simulink model "task4_rfj"  (R2022b)
settings: Solver=VariableStepAuto  StartTime=0.0  StopTime=param.T  FixedStep=0.01  MaxStep=0.01  RelTol=1e-3
undefined symbols (not defined in the file or in its folder): param
settings Model: Creator=15043  LastModifiedBy=15043
settings SolverCC: AlgebraicLoopSolver=TrustRegion
settings DebuggingCC: ArithmeticOperatorsInVariantConditions=warning
settings SFSimCC: CustomCodeUndefinedFunction=UseInterfaceOnly

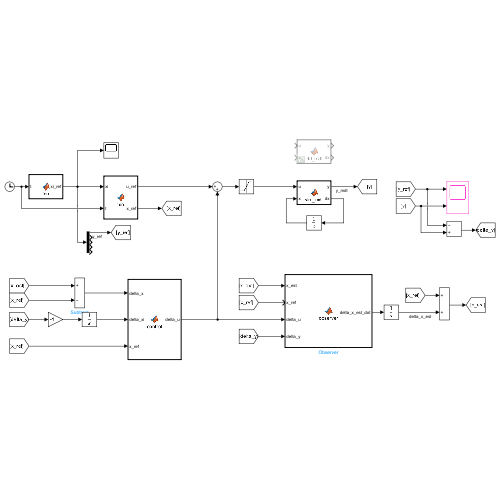
[thumbnail: Simulink's stored preview of the top-level diagram]
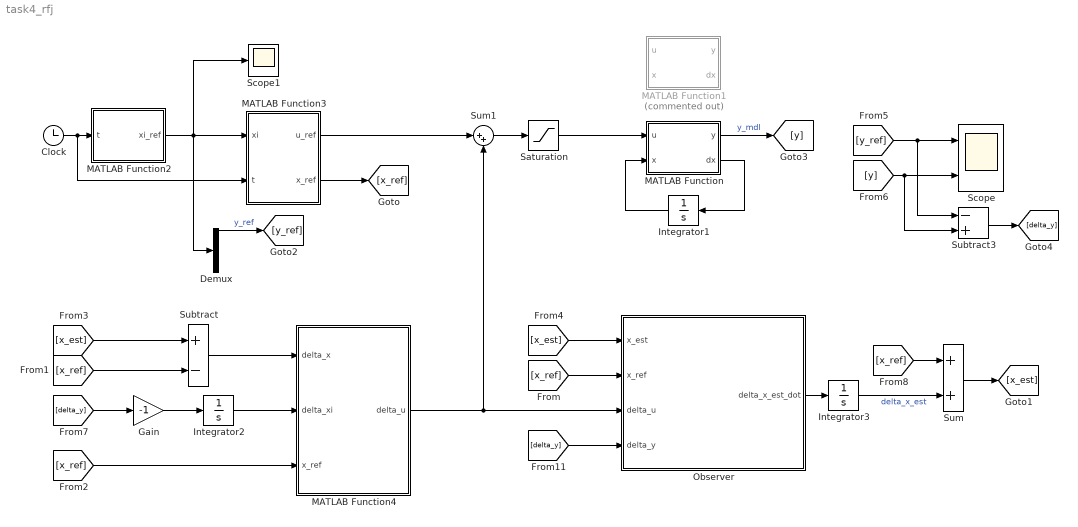
== system task4_rfj ==
  Clock : Clock
  Demux : Demux  Outputs=5
  Gain : Gain  Gain=-1
  Integrator1 : Integrator  InitialCondition=param.x0
  Integrator2 : Integrator
  Integrator3 : Integrator  InitialCondition=param.delta_x_est0
  MATLAB Function : MATLAB Function  TreatAsAtomicUnit=on
  MATLAB Function1 : MATLAB Function  Commented=on  TreatAsAtomicUnit=on
  MATLAB Function2 : MATLAB Function  TreatAsAtomicUnit=on
  MATLAB Function3 : MATLAB Function  TreatAsAtomicUnit=on
  MATLAB Function4 : MATLAB Function  TreatAsAtomicUnit=on
  Observer : MATLAB Function  TreatAsAtomicUnit=on
  Saturation : Saturate  UpperLimit=10  LowerLimit=-10
  Scope : Scope  NumInputPorts=2
  Scope1 : Scope
  Subtract : Sum  Inputs=+-
  Subtract3 : Sum  Inputs=-+
  Sum : Sum
  Sum1 : Sum  Inputs=|++
  wires:
  MATLAB Function/2(dx) -> Integrator1/1
  Integrator1/1 -> MATLAB Function/2(x)
  MATLAB Function/1(y) -> [y]  "y_mdl"
  Clock/1 -> MATLAB Function3/2(t), MATLAB Function2/1(t)
  Demux/1 -> [y_ref]  "y_ref"
  MATLAB Function2/1(xi_ref) -> Scope1/1, Demux/1, MATLAB Function3/1(xi)
  MATLAB Function3/2(x_ref) -> [x_ref]
  Subtract/1 -> MATLAB Function4/1(delta_x)
  Gain/1 -> Integrator2/1
  Integrator2/1 -> MATLAB Function4/2(delta_xi)
  MATLAB Function4/1(delta_u) -> Sum1/2, Observer/3(delta_u)
  MATLAB Function3/1(u_ref) -> Sum1/1
  Observer/1(delta_x_est_dot) -> Integrator3/1
  Sum/1 -> [x_est]
  Integrator3/1 -> Sum/2  "delta_x_est"
  [x_ref] -> Observer/2(x_ref)
  [x_ref] -> Subtract/2
  [x_ref] -> MATLAB Function4/3(x_ref)
  [x_est] -> Observer/1(x_est)
  [y_ref] -> Subtract3/1, Scope/1
  [y] -> Scope/2, Subtract3/2
  Subtract3/1 -> [delta_y]
  [delta_y] -> Observer/4(delta_y)
  [delta_y] -> Gain/1
  [x_ref] -> Sum/1
  Sum1/1 -> Saturation/1
  Saturation/1 -> MATLAB Function/1(u)
  [x_est] -> Subtract/1

== matlab function task4_rfj/MATLAB Function1 ==
  data: y output; dx output; u input; x input; param parameter
function [y, dx]= ctrl_mdl(u, x, param)

    g = param.g;
%     l_c = param.l_c;
%     l_ax = param.l_ax;
%     l_ay = param.l_ay;
%     k_f = param.k_t;
%     s_0 = param.s_0;
    k_r = param.kr;
    m_B1 = param.m_B1;
    m_B2 = param.m_B2;
%     l_B1 = param.l_B1;
%     l_B2 = param.l_B2;
    J_Pzz = param.J_Pzz;
    d_P = param.d_P;
    R_m = param.R_m;
    k_b = param.k_b;
    k_m = param.k_m;
    K_g = param.K_g;
    eta_g = param.eta_g;
    eta_m = param.eta_m;
    %nu = param.nu;
    J_Bzz = param.J_Bzz;
    l_G = param.l_G;



    x1 = x(1);
    x2 = x(2);
    x3 = x(3);
    x4 = x(4);
    
    f1 = x2;
    f3 = x4;
    f2 = (-(R_m*d_P + K_g*eta_g*eta_m*k_b*k_m)/(J_Pzz*R_m))*x2 + (k_r/J_Pzz)*x3;
    f4 = ((g*l_G*(m_B1 + m_B2))/J_Bzz)*sin(x1 + x3) + (x2*(R_m*d_P + K_g*eta_g*eta_m*k_b*k_m))/(J_Pzz*R_m) - (k_r*x3*(J_Bzz + J_Pzz))/(J_Bzz*J_Pzz);

    f = [f1; f2; f3; f4];
    
    g = [0;
        (K_g*eta_g*eta_m*k_b)/(J_Pzz*R_m);
        0;
        -(K_g*eta_g*eta_m*k_b)/(J_Pzz*R_m)];
    
    dx = f + g*u;
    y = x1 + x3;

end

== matlab function task4_rfj/MATLAB Function ==
  data: y output; dx output; u input; x input; param parameter
function [y, dx]= sim_mdl(u, x, param)

    g = param.g;
    l_c = param.l_c;
    l_ax = param.l_ax;
    l_ay = param.l_ay;
    k_f = param.k_t;
    s_0 = param.s_0;
    m_B1 = param.m_B1;
    m_B2 = param.m_B2;
%     l_B1 = param.l_B1;
%     l_B2 = param.l_B2;
    J_Pzz = param.J_Pzz;
    d_P = param.d_P;
    R_m = param.R_m;
    k_b = param.k_b;
    k_m = param.k_m;
    K_g = param.K_g;
    eta_g = param.eta_g;
    eta_m = param.eta_m;
    %nu = param.nu;
    J_Bzz = param.J_Bzz;
    l_G = param.l_G;


    x1 = x(1);
    x2 = x(2);
    x3 = x(3);
    x4 = x(4);
    
    f1 = x2;
    f3 = x4;
    f2 =  (-((k_f*l_ax*l_c*s_0)/((l_ax - l_c*cos(x3))^2 + (l_ay + l_c*sin(x3))^2)^(1/2) - 2*k_f*l_ax*l_c + (k_f*l_ax*l_c*s_0)/((l_ax - l_c*cos(x3))^2 + (l_ay - l_c*sin(x3))^2)^(1/2))/J_Pzz)*sin(x3) + (-((k_f*l_ay*l_c*s_0)/((l_ax - l_c*cos(x3))^2 + (l_ay + l_c*sin(x3))^2)^(1/2) - (k_f*l_ay*l_c*s_0)/((l_ax - l_c*cos(x3))^2 + (l_ay - l_c*sin(x3))^2)^(1/2))/J_Pzz)*cos(x3) + (-(d_P + (K_g*eta_g*eta_m*k_b*k_m)/R_m)/J_Pzz)*x2;
    f4 =  ((g*l_G*m_B1 + g*l_G*m_B2)/J_Bzz)*sin(x1 + x3) + (((J_Bzz*((k_f*l_ax*l_c*s_0)/((l_ax - l_c*cos(x3))^2 + (l_ay + l_c*sin(x3))^2)^(1/2) - 2*k_f*l_ax*l_c + (k_f*l_ax*l_c*s_0)/((l_ax - l_c*cos(x3))^2 + (l_ay - l_c*sin(x3))^2)^(1/2)))/J_Pzz - 2*k_f*l_ax*l_c + (k_f*l_ax*l_c*s_0)/((l_ax - l_c*cos(x3))^2 + (l_ay + l_c*sin(x3))^2)^(1/2) + (k_f*l_ax*l_c*s_0)/((l_ax - l_c*cos(x3))^2 + (l_ay - l_c*sin(x3))^2)^(1/2))/J_Bzz)*sin(x3) + (((J_Bzz*((k_f*l_ay*l_c*s_0)/((l_ax - l_c*cos(x3))^2 + (l_ay + l_c*sin(x3))^2)^(1/2) - (k_f*l_ay*l_c*s_0)/((l_ax - l_c*cos(x3))^2 + (l_ay - l_c*sin(x3))^2)^(1/2)))/J_Pzz + (k_f*l_ay*l_c*s_0)/((l_ax - l_c*cos(x3))^2 + (l_ay + l_c*sin(x3))^2)^(1/2) - (k_f*l_ay*l_c*s_0)/((l_ax - l_c*cos(x3))^2 + (l_ay - l_c*sin(x3))^2)^(1/2))/J_Bzz)*cos(x3) + (d_P*x2 + (K_g*eta_g*eta_m*k_b*k_m*x2)/R_m)/J_Pzz;

    f = [f1; f2; f3; f4];
    
    g = [0;
        (K_g*eta_g*eta_m*k_b)/(J_Pzz*R_m);
        0;
        -(K_g*eta_g*eta_m*k_b)/(J_Pzz*R_m)];
    
    dx = f + g*u;
    y = x1 + x3;

end

== matlab function task4_rfj/MATLAB Function2 ==
  data: t input; xi_ref output; param parameter
function xi_ref = fcn(t, param)

    beta = param.beta;
    lambda_R0 = param.lambda_R0;
    lambda_R1 = param.lambda_R1;
    t_0 = param.t_0;
    t_1 = param.t_1;

    xi_ref = zeros(5, 1);
    if t<t_0
        xi_ref(1) = lambda_R0;
    elseif t>=t_1
        xi_ref(1) = lambda_R1;
    else
        xi_ref = zeros(5,1);
        xi_ref(1) = lambda_R0 + ((t - t_0)^9*(70*lambda_R0 - 70*lambda_R1))/(t_0 - t_1)^9 + ((t - t_0)^5*(126*lambda_R0 - 126*lambda_R1))/(t_0 - t_1)^5 + ((t - t_0)^8*(315*lambda_R0 - 315*lambda_R1))/(t_0 - t_1)^8 + ((t - t_0)^6*(420*lambda_R0 - 420*lambda_R1))/(t_0 - t_1)^6 + ((t - t_0)^7*(540*lambda_R0 - 540*lambda_R1))/(t_0 - t_1)^7;
        xi_ref(2) = (9*(t - t_0)^8*(70*lambda_R0 - 70*lambda_R1))/(t_0 - t_1)^9 + (5*(t - t_0)^4*(126*lambda_R0 - 126*lambda_R1))/(t_0 - t_1)^5 + (8*(t - t_0)^7*(315*lambda_R0 - 315*lambda_R1))/(t_0 - t_1)^8 + (6*(t - t_0)^5*(420*lambda_R0 - 420*lambda_R1))/(t_0 - t_1)^6 + (7*(t - t_0)^6*(540*lambda_R0 - 540*lambda_R1))/(t_0 - t_1)^7;
        xi_ref(3) = (72*(t - t_0)^7*(70*lambda_R0 - 70*lambda_R1))/(t_0 - t_1)^9 + (20*(t - t_0)^3*(126*lambda_R0 - 126*lambda_R1))/(t_0 - t_1)^5 + (56*(t - t_0)^6*(315*lambda_R0 - 315*lambda_R1))/(t_0 - t_1)^8 + (30*(t - t_0)^4*(420*lambda_R0 - 420*lambda_R1))/(t_0 - t_1)^6 + (42*(t - t_0)^5*(540*lambda_R0 - 540*lambda_R1))/(t_0 - t_1)^7;
        xi_ref(4) = (504*(t - t_0)^6*(70*lambda_R0 - 70*lambda_R1))/(t_0 - t_1)^9 + (60*(t - t_0)^2*(126*lambda_R0 - 126*lambda_R1))/(t_0 - t_1)^5 + (336*(t - t_0)^5*(315*lambda_R0 - 315*lambda_R1))/(t_0 - t_1)^8 + (120*(t - t_0)^3*(420*lambda_R0 - 420*lambda_R1))/(t_0 - t_1)^6 + (210*(t - t_0)^4*(540*lambda_R0 - 540*lambda_R1))/(t_0 - t_1)^7;
        xi_ref(5) = (60*(2*t - 2*t_0)*(126*lambda_R0 - 126*lambda_R1))/(t_0 - t_1)^5 + (3024*(t - t_0)^5*(70*lambda_R0 - 70*lambda_R1))/(t_0 - t_1)^9 + (1680*(t - t_0)^4*(315*lambda_R0 - 315*lambda_R1))/(t_0 - t_1)^8 + (360*(t - t_0)^2*(420*lambda_R0 - 420*lambda_R1))/(t_0 - t_1)^6 + (840*(t - t_0)^3*(540*lambda_R0 - 540*lambda_R1))/(t_0 - t_1)^7;
    end
end

== matlab function task4_rfj/MATLAB Function3 ==
  data: xi input; u_ref output; param parameter; x_ref output; t input
function [u_ref, x_ref] = fcn(xi, param, t)
    
    g = param.g;
%     l_c = param.l_c;
%     l_ax = param.l_ax;
%     l_ay = param.l_ay;
%     k_f = param.k_t;
%     s_0 = param.s_0;
    k_r = param.kr;
    m_B1 = param.m_B1;
    m_B2 = param.m_B2;
%     l_B1 = param.l_B1;
%     l_B2 = param.l_B2;
    J_Pzz = param.J_Pzz;
    d_P = param.d_P;
    R_m = param.R_m;
    k_b = param.k_b;
    k_m = param.k_m;
    K_g = param.K_g;
    eta_g = param.eta_g;
    eta_m = param.eta_m;
    %nu = param.nu;
    J_Bzz = param.J_Bzz;
    l_G = param.l_G;

    xi1 = xi(1);
    xi2 = xi(2);
    xi3 = xi(3);
    xi4 = xi(4);
    xi5 = xi(5);
    
    x_ref = [xi1 - (sin(xi1)*(g*l_G*m_B1 + g*l_G*m_B2))/k_r + (J_Bzz*xi3)/k_r;
               xi2 + (J_Bzz*xi4)/k_r - (xi2*cos(xi1)*(g*l_G*m_B1 + g*l_G*m_B2))/k_r;
                (sin(xi1)*(g*l_G*m_B1 + g*l_G*m_B2))/k_r - (J_Bzz*xi3)/k_r;
                (xi2*cos(xi1)*(g*l_G*m_B1 + g*l_G*m_B2))/k_r - (J_Bzz*xi4)/k_r;];   

    u_ref = (J_Bzz*J_Pzz*R_m*(xi5 - ((g*l_G*m_B1*cos(xi1) - k_r + g*l_G*m_B2*cos(xi1))*(((R_m*d_P + K_g*eta_g*eta_m*k_b*k_m)*(xi2 + (J_Bzz*xi4)/k_r - (xi2*cos(xi1)*(g*l_G*m_B1 + g*l_G*m_B2))/k_r))/(J_Pzz*R_m) + (g*l_G*sin(xi1)*(m_B1 + m_B2))/J_Bzz - (k_r*((sin(xi1)*(g*l_G*m_B1 + g*l_G*m_B2))/k_r - (J_Bzz*xi3)/k_r)*(J_Bzz + J_Pzz))/(J_Bzz*J_Pzz)))/J_Bzz + (g*l_G*xi2*sin(xi1)*(m_B1 + m_B2)*(xi2 + (J_Bzz*xi4)/k_r - (xi2*cos(xi1)*(g*l_G*m_B1 + g*l_G*m_B2))/k_r))/J_Bzz - (g*l_G*xi2*sin(xi1)*(m_B1 + m_B2)*((J_Bzz*xi4)/k_r - (xi2*cos(xi1)*(g*l_G*m_B1 + g*l_G*m_B2))/k_r))/J_Bzz + (g*l_G*cos(xi1)*(m_B1 + m_B2)*(R_m*d_P*(xi2 + (J_Bzz*xi4)/k_r - (xi2*cos(xi1)*(g*l_G*m_B1 + g*l_G*m_B2))/k_r) - R_m*k_r*((sin(xi1)*(g*l_G*m_B1 + g*l_G*m_B2))/k_r - (J_Bzz*xi3)/k_r) + K_g*eta_g*eta_m*k_b*k_m*(xi2 + (J_Bzz*xi4)/k_r - (xi2*cos(xi1)*(g*l_G*m_B1 + g*l_G*m_B2))/k_r)))/(J_Bzz*J_Pzz*R_m)))/(K_g*eta_g*eta_m*k_b*k_r);
%    if t>param.t_1
%        u_ref = 0;
%    end
end

== matlab function task4_rfj/MATLAB Function4 ==
  data: delta_x input; delta_u output; delta_xi input; x_ref input; param parameter
function delta_u = control(delta_x, delta_xi, x_ref, param)

    g = param.g;
%     l_c = param.l_c;
%     l_ax = param.l_ax;
%     l_ay = param.l_ay;
%     k_f = param.k_t;
%     s_0 = param.s_0;
    k_r = param.kr;
    m_B1 = param.m_B1;
    m_B2 = param.m_B2;
%     l_B1 = param.l_B1;
%     l_B2 = param.l_B2;
    J_Pzz = param.J_Pzz;
    d_P = param.d_P;
    R_m = param.R_m;
    k_b = param.k_b;
    k_m = param.k_m;
    K_g = param.K_g;
    eta_g = param.eta_g;
    eta_m = param.eta_m;
    %nu = param.nu;
    J_Bzz = param.J_Bzz;
    l_G = param.l_G;
    p0 = param.p01;
    p1 = param.p11;
    p2 = param.p21;
    p3 = param.p31;
    p4 = param.p41;


    x1 = x_ref(1);
    x2 = x_ref(2);
    x3 = x_ref(3);
    x4 = x_ref(4);

%     k = [(J_Bzz^3*J_Pzz^5*R_m^5*((g*l_G*cos(x1 + x3)*(m_B1 + m_B2)*((K_g^4*eta_g^4*eta_m^4*k_b^4*k_r^3)/(J_Bzz^2*J_Pzz^5*R_m^4) - (K_g^4*eta_g^4*eta_m^4*k_b^4*k_r^2*((k_r*(J_Bzz + J_Pzz))/(J_Bzz*J_Pzz) - (g*l_G*cos(x1 + x3)*(m_B1 + m_B2))/J_Bzz))/(J_Bzz^2*J_Pzz^4*R_m^4)))/J_Bzz + (K_g^4*eta_g^4*eta_m^4*k_b^4*k_r^2)/(J_Bzz^2*J_Pzz^4*R_m^4) + (K_g^4*eta_g^4*eta_m^4*g*k_b^4*k_r^2*l_G*cos(x1 + x3)*(m_B1 + m_B2))/(J_Bzz^3*J_Pzz^4*R_m^4)))/(K_g^5*eta_g^5*eta_m^5*k_b^5*k_r^3), (J_Bzz^3*J_Pzz^5*R_m^5*(((R_m*d_P + K_g*eta_g*eta_m*k_b*k_m)*((K_g^4*eta_g^4*eta_m^4*k_b^4*k_r^3)/(J_Bzz^2*J_Pzz^5*R_m^4) - (K_g^4*eta_g^4*eta_m^4*k_b^4*k_r^2*((k_r*(J_Bzz + J_Pzz))/(J_Bzz*J_Pzz) - (g*l_G*cos(x1 + x3)*(m_B1 + m_B2))/J_Bzz))/(J_Bzz^2*J_Pzz^4*R_m^4)))/(J_Pzz*R_m) + (K_g^4*eta_g^4*eta_m^4*k_b^4*k_r^2)/(J_Bzz^2*J_Pzz^4*R_m^4) + (K_g^4*eta_g^4*eta_m^4*g*k_b^4*k_r^2*l_G*cos(x1 + x3)*(m_B1 + m_B2))/(J_Bzz^3*J_Pzz^4*R_m^4) - (K_g^4*eta_g^4*eta_m^4*g*k_b^4*k_r^2*l_G*cos(x1 + x3)*(m_B1 + m_B2)*(R_m*d_P + K_g*eta_g*eta_m*k_b*k_m))/(J_Bzz^3*J_Pzz^5*R_m^5)))/(K_g^5*eta_g^5*eta_m^5*k_b^5*k_r^3), (J_Bzz^3*J_Pzz^5*R_m^5*((K_g^4*eta_g^4*eta_m^4*k_b^4*k_r^2)/(J_Bzz^2*J_Pzz^4*R_m^4) - ((k_r*(J_Bzz + J_Pzz))/(J_Bzz*J_Pzz) - (g*l_G*cos(x1 + x3)*(m_B1 + m_B2))/J_Bzz)*((K_g^4*eta_g^4*eta_m^4*k_b^4*k_r^3)/(J_Bzz^2*J_Pzz^5*R_m^4) - (K_g^4*eta_g^4*eta_m^4*k_b^4*k_r^2*((k_r*(J_Bzz + J_Pzz))/(J_Bzz*J_Pzz) - (g*l_G*cos(x1 + x3)*(m_B1 + m_B2))/J_Bzz))/(J_Bzz^2*J_Pzz^4*R_m^4)) + (K_g^4*eta_g^4*eta_m^4*k_b^4*k_r^3)/(J_Bzz^2*J_Pzz^5*R_m^4) - (K_g^4*eta_g^4*eta_m^4*k_b^4*k_r^2*((k_r*(J_Bzz + J_Pzz))/(J_Bzz*J_Pzz) - (g*l_G*cos(x1 + x3)*(m_B1 + m_B2))/J_Bzz))/(J_Bzz^2*J_Pzz^4*R_m^4) + (K_g^4*eta_g^4*eta_m^4*g*k_b^4*k_r^3*l_G*cos(x1 + x3)*(m_B1 + m_B2))/(J_Bzz^3*J_Pzz^5*R_m^4)))/(K_g^5*eta_g^5*eta_m^5*k_b^5*k_r^3), (J_Bzz^3*J_Pzz^5*R_m^5*((K_g^4*eta_g^4*eta_m^4*k_b^4*k_r^2)/(J_Bzz^2*J_Pzz^4*R_m^4) + (K_g^4*eta_g^4*eta_m^4*k_b^4*k_r^3)/(J_Bzz^2*J_Pzz^5*R_m^4) - (K_g^4*eta_g^4*eta_m^4*k_b^4*k_r^2*((k_r*(J_Bzz + J_Pzz))/(J_Bzz*J_Pzz) - (g*l_G*cos(x1 + x3)*(m_B1 + m_B2))/J_Bzz))/(J_Bzz^2*J_Pzz^4*R_m^4)))/(K_g^5*eta_g^5*eta_m^5*k_b^5*k_r^3), -(J_Bzz*J_Pzz*R_m)/(K_g*eta_g*eta_m*k_b*k_r)];
%    k = [-(p1*J_Bzz^2 + p3*J_Bzz*g*l_G*m_B1*cos(x1 + x3) + p3*J_Bzz*g*l_G*m_B2*cos(x1 + x3) + g^2*l_G^2*m_B1^2*cos(x1 + x3)^2 + 2*g^2*l_G^2*m_B1*m_B2*cos(x1 + x3)^2 + g^2*l_G^2*m_B2^2*cos(x1 + x3)^2 - k_r*g*l_G*m_B1*cos(x1 + x3) - k_r*g*l_G*m_B2*cos(x1 + x3))/J_Bzz^2, -(J_Bzz*J_Pzz*R_m*p2 - R_m*d_P*k_r - K_g*eta_g*eta_m*k_b*k_m*k_r + J_Pzz*R_m*g*l_G*m_B1*p4*cos(x1 + x3) + J_Pzz*R_m*g*l_G*m_B2*p4*cos(x1 + x3))/(J_Bzz*J_Pzz*R_m), -(J_Pzz*p1*J_Bzz^2 + J_Pzz*p3*J_Bzz*g*l_G*m_B1*cos(x1 + x3) + J_Pzz*p3*J_Bzz*g*l_G*m_B2*cos(x1 + x3) + J_Bzz*k_r^2 - J_Pzz*p3*J_Bzz*k_r + J_Pzz*g^2*l_G^2*m_B1^2*cos(x1 + x3)^2 + 2*J_Pzz*g^2*l_G^2*m_B1*m_B2*cos(x1 + x3)^2 + J_Pzz*g^2*l_G^2*m_B2^2*cos(x1 + x3)^2 - 2*J_Pzz*g*k_r*l_G*m_B1*cos(x1 + x3) - 2*J_Pzz*g*k_r*l_G*m_B2*cos(x1 + x3) + J_Pzz*k_r^2)/(J_Bzz^2*J_Pzz), -(J_Bzz*p2 - k_r*p4 + g*l_G*m_B1*p4*cos(x1 + x3) + g*l_G*m_B2*p4*cos(x1 + x3))/J_Bzz, p0];
    k = [(J_Bzz*J_Pzz*R_m*(p1 + (g*l_G*p3*cos(x1 + x3)*(m_B1 + m_B2))/J_Bzz + (g*l_G*cos(x1 + x3)*(m_B1 + m_B2)*(k_r/J_Pzz - (k_r*(J_Bzz + J_Pzz))/(J_Bzz*J_Pzz) + (g*l_G*cos(x1 + x3)*(m_B1 + m_B2))/J_Bzz))/J_Bzz))/(K_g*eta_g*eta_m*k_b*k_r), (J_Bzz*J_Pzz*R_m*(p2 + ((R_m*d_P + K_g*eta_g*eta_m*k_b*k_m)*(k_r/J_Pzz - (k_r*(J_Bzz + J_Pzz))/(J_Bzz*J_Pzz) + (g*l_G*cos(x1 + x3)*(m_B1 + m_B2))/J_Bzz))/(J_Pzz*R_m) + (g*l_G*p4*cos(x1 + x3)*(m_B1 + m_B2))/J_Bzz - (g*l_G*cos(x1 + x3)*(m_B1 + m_B2)*(R_m*d_P + K_g*eta_g*eta_m*k_b*k_m))/(J_Bzz*J_Pzz*R_m)))/(K_g*eta_g*eta_m*k_b*k_r), (J_Bzz*J_Pzz*R_m*(p1 - ((k_r*(J_Bzz + J_Pzz))/(J_Bzz*J_Pzz) - (g*l_G*cos(x1 + x3)*(m_B1 + m_B2))/J_Bzz)*(k_r/J_Pzz - (k_r*(J_Bzz + J_Pzz))/(J_Bzz*J_Pzz) + (g*l_G*cos(x1 + x3)*(m_B1 + m_B2))/J_Bzz) + p3*(k_r/J_Pzz - (k_r*(J_Bzz + J_Pzz))/(J_Bzz*J_Pzz) + (g*l_G*cos(x1 + x3)*(m_B1 + m_B2))/J_Bzz) + (g*k_r*l_G*cos(x1 + x3)*(m_B1 + m_B2))/(J_Bzz*J_Pzz)))/(K_g*eta_g*eta_m*k_b*k_r), (J_Bzz*J_Pzz*R_m*(p2 + p4*(k_r/J_Pzz - (k_r*(J_Bzz + J_Pzz))/(J_Bzz*J_Pzz) + (g*l_G*cos(x1 + x3)*(m_B1 + m_B2))/J_Bzz)))/(K_g*eta_g*eta_m*k_b*k_r), -(J_Bzz*J_Pzz*R_m*p0)/(K_g*eta_g*eta_m*k_b*k_r)];
    delta_u = -k*[delta_x; delta_xi];

end

== matlab function task4_rfj/Observer ==
  data: x_est input; x_ref input; delta_u input; delta_y input; delta_x_est_dot output; param parameter
function delta_x_est_dot  = observer(x_est, x_ref, delta_u, delta_y, param)
    
    g = param.g;
%     l_c = param.l_c;
%     l_ax = param.l_ax;
%     l_ay = param.l_ay;
%     k_f = param.k_t;
%     s_0 = param.s_0;
    k_r = param.kr;
    m_B1 = param.m_B1;
    m_B2 = param.m_B2;
%     l_B1 = param.l_B1;
%     l_B2 = param.l_B2;
    J_Pzz = param.J_Pzz;
    d_P = param.d_P;
    R_m = param.R_m;
    k_b = param.k_b;
    k_m = param.k_m;
    K_g = param.K_g;
    eta_g = param.eta_g;
    eta_m = param.eta_m;
    %nu = param.nu;
    J_Bzz = param.J_Bzz;
    l_G = param.l_G;

    p0 = param.p02;
    p1 = param.p12;
    p2 = param.p22; 
    p3 = param.p32;

    x1 = x_est(1);
    x2 = x_est(2);
    x3 = x_est(3);
    x4 = x_est(4);
    
    f1 = x2;
    f3 = x4;
    f2 = (-(R_m*d_P + K_g*eta_g*eta_m*k_b*k_m)/(J_Pzz*R_m))*x2 + (k_r/J_Pzz)*x3;
    f4 = ((g*l_G*(m_B1 + m_B2))/J_Bzz)*sin(x1 + x3) + (x2*(R_m*d_P + K_g*eta_g*eta_m*k_b*k_m))/(J_Pzz*R_m) - (k_r*x3*(J_Bzz + J_Pzz))/(J_Bzz*J_Pzz);

    f_x_est = [f1; f2; f3; f4];


    x1 = x_ref(1);
    x2 = x_ref(2);
    x3 = x_ref(3);
    x4 = x_ref(4);
    
    f1 = x2;
    f3 = x4;
    f2 = (-(R_m*d_P + K_g*eta_g*eta_m*k_b*k_m)/(J_Pzz*R_m))*x2 + (k_r/J_Pzz)*x3;
    f4 = ((g*l_G*(m_B1 + m_B2))/J_Bzz)*sin(x1 + x3) + (x2*(R_m*d_P + K_g*eta_g*eta_m*k_b*k_m))/(J_Pzz*R_m) - (k_r*x3*(J_Bzz + J_Pzz))/(J_Bzz*J_Pzz);

    f_x_ref = [f1; f2; f3; f4];
    
    gx = [0;
        (K_g*eta_g*eta_m*k_b)/(J_Pzz*R_m);
        0;
        -(K_g*eta_g*eta_m*k_b)/(J_Pzz*R_m)];
    
%     l = [(J_Bzz^2*(k_r/J_Bzz - k_r^2/(J_Bzz*J_Pzz) + ((R_m*d_P + K_g*eta_g*eta_m*k_b*k_m)*(k_r^2/(J_Bzz*J_Pzz) - ((R_m*d_P + K_g*eta_g*eta_m*k_b*k_m)^2*k_r)/(J_Bzz*J_Pzz^2*R_m^2)))/(J_Pzz*R_m) - (k_r*(R_m*d_P + K_g*eta_g*eta_m*k_b*k_m))/(J_Bzz*J_Pzz*R_m) + (k_r^2*(R_m*d_P + K_g*eta_g*eta_m*k_b*k_m))/(J_Bzz*J_Pzz^2*R_m) + (k_r*(R_m*d_P + K_g*eta_g*eta_m*k_b*k_m)^2)/(J_Bzz*J_Pzz^2*R_m^2)))/k_r^2;
%         (J_Bzz^2*(k_r/J_Bzz - k_r^2/(J_Bzz*J_Pzz) + (k_r*((k_r*((k_r*(J_Bzz + J_Pzz))/(J_Bzz*J_Pzz) - (g*l_G*cos(x1 + x3)*(m_B1 + m_B2))/J_Bzz))/J_Bzz - (k_r*(R_m*d_P + K_g*eta_g*eta_m*k_b*k_m)^2)/(J_Bzz*J_Pzz^2*R_m^2) + (g*k_r*l_G*cos(x1 + x3)*(m_B1 + m_B2))/J_Bzz^2))/J_Pzz - ((((R_m*d_P + K_g*eta_g*eta_m*k_b*k_m)*(k_r^2/(J_Bzz*J_Pzz) - ((R_m*d_P + K_g*eta_g*eta_m*k_b*k_m)^2*k_r)/(J_Bzz*J_Pzz^2*R_m^2)))/(J_Pzz*R_m) + (k_r^2*(R_m*d_P + K_g*eta_g*eta_m*k_b*k_m))/(J_Bzz*J_Pzz^2*R_m))*(R_m*d_P + K_g*eta_g*eta_m*k_b*k_m))/(J_Pzz*R_m) + ((R_m*d_P + K_g*eta_g*eta_m*k_b*k_m)*(k_r^2/(J_Bzz*J_Pzz) - ((R_m*d_P + K_g*eta_g*eta_m*k_b*k_m)^2*k_r)/(J_Bzz*J_Pzz^2*R_m^2)))/(J_Pzz*R_m) - (k_r*(R_m*d_P + K_g*eta_g*eta_m*k_b*k_m))/(J_Bzz*J_Pzz*R_m) + (k_r^2*(R_m*d_P + K_g*eta_g*eta_m*k_b*k_m))/(J_Bzz*J_Pzz^2*R_m) + (k_r*(R_m*d_P + K_g*eta_g*eta_m*k_b*k_m)^2)/(J_Bzz*J_Pzz^2*R_m^2)))/k_r^2;
%         -(J_Bzz^2*(k_r/J_Bzz - (k_r*((k_r*(J_Bzz + J_Pzz))/(J_Bzz*J_Pzz) - (g*l_G*cos(x1 + x3)*(m_B1 + m_B2))/J_Bzz))/J_Bzz + ((R_m*d_P + K_g*eta_g*eta_m*k_b*k_m)*(k_r^2/(J_Bzz*J_Pzz) - ((R_m*d_P + K_g*eta_g*eta_m*k_b*k_m)^2*k_r)/(J_Bzz*J_Pzz^2*R_m^2)))/(J_Pzz*R_m) - (k_r*(R_m*d_P + K_g*eta_g*eta_m*k_b*k_m))/(J_Bzz*J_Pzz*R_m) + (k_r*(R_m*d_P + K_g*eta_g*eta_m*k_b*k_m)^2)/(J_Bzz*J_Pzz^2*R_m^2) - (g*k_r*l_G*cos(x1 + x3)*(m_B1 + m_B2))/J_Bzz^2 + (k_r*((k_r*(J_Bzz + J_Pzz))/(J_Bzz*J_Pzz) - (g*l_G*cos(x1 + x3)*(m_B1 + m_B2))/J_Bzz)*(R_m*d_P + K_g*eta_g*eta_m*k_b*k_m))/(J_Bzz*J_Pzz*R_m) + (g*k_r*l_G*cos(x1 + x3)*(m_B1 + m_B2)*(R_m*d_P + K_g*eta_g*eta_m*k_b*k_m))/(J_Bzz^2*J_Pzz*R_m)))/k_r^2;
%         -(J_Bzz^2*(k_r/J_Bzz + ((k_r*(J_Bzz + J_Pzz))/(J_Bzz*J_Pzz) - (g*l_G*cos(x1 + x3)*(m_B1 + m_B2))/J_Bzz)*((k_r*((k_r*(J_Bzz + J_Pzz))/(J_Bzz*J_Pzz) - (g*l_G*cos(x1 + x3)*(m_B1 + m_B2))/J_Bzz))/J_Bzz - (k_r*(R_m*d_P + K_g*eta_g*eta_m*k_b*k_m)^2)/(J_Bzz*J_Pzz^2*R_m^2) + (g*k_r*l_G*cos(x1 + x3)*(m_B1 + m_B2))/J_Bzz^2) - (k_r*((k_r*(J_Bzz + J_Pzz))/(J_Bzz*J_Pzz) - (g*l_G*cos(x1 + x3)*(m_B1 + m_B2))/J_Bzz))/J_Bzz - ((((R_m*d_P + K_g*eta_g*eta_m*k_b*k_m)*(k_r^2/(J_Bzz*J_Pzz) - ((R_m*d_P + K_g*eta_g*eta_m*k_b*k_m)^2*k_r)/(J_Bzz*J_Pzz^2*R_m^2)))/(J_Pzz*R_m) + (k_r^2*(R_m*d_P + K_g*eta_g*eta_m*k_b*k_m))/(J_Bzz*J_Pzz^2*R_m))*(R_m*d_P + K_g*eta_g*eta_m*k_b*k_m))/(J_Pzz*R_m) + ((R_m*d_P + K_g*eta_g*eta_m*k_b*k_m)*(k_r^2/(J_Bzz*J_Pzz) - ((R_m*d_P + K_g*eta_g*eta_m*k_b*k_m)^2*k_r)/(J_Bzz*J_Pzz^2*R_m^2)))/(J_Pzz*R_m) - (k_r*(R_m*d_P + K_g*eta_g*eta_m*k_b*k_m))/(J_Bzz*J_Pzz*R_m) + (k_r*(R_m*d_P + K_g*eta_g*eta_m*k_b*k_m)^2)/(J_Bzz*J_Pzz^2*R_m^2) - (g*k_r*l_G*cos(x1 + x3)*(m_B1 + m_B2))/J_Bzz^2 + (g*l_G*cos(x1 + x3)*(m_B1 + m_B2)*(k_r^2/(J_Bzz*J_Pzz) - ((R_m*d_P + K_g*eta_g*eta_m*k_b*k_m)^2*k_r)/(J_Bzz*J_Pzz^2*R_m^2)))/J_Bzz + (k_r*((k_r*(J_Bzz + J_Pzz))/(J_Bzz*J_Pzz) - (g*l_G*cos(x1 + x3)*(m_B1 + m_B2))/J_Bzz)*(R_m*d_P + K_g*eta_g*eta_m*k_b*k_m))/(J_Bzz*J_Pzz*R_m) + (g*k_r*l_G*cos(x1 + x3)*(m_B1 + m_B2)*(R_m*d_P + K_g*eta_g*eta_m*k_b*k_m))/(J_Bzz^2*J_Pzz*R_m)))/k_r^2;];
    l = zeros(4,1);
    l(1,1) = (J_Bzz*(p1 - p3*(k_r/J_Pzz - (R_m*d_P + K_g*eta_g*eta_m*k_b*k_m)^2/(J_Pzz^2*R_m^2)) + ((k_r/J_Pzz - (R_m*d_P + K_g*eta_g*eta_m*k_b*k_m)^2/(J_Pzz^2*R_m^2))*(R_m*d_P + K_g*eta_g*eta_m*k_b*k_m))/(J_Pzz*R_m) + (k_r*(R_m*d_P + K_g*eta_g*eta_m*k_b*k_m))/(J_Pzz^2*R_m) - (p2*(R_m*d_P + K_g*eta_g*eta_m*k_b*k_m))/(J_Pzz*R_m)))/k_r;
    l(2,1) = -(J_Bzz*(p2*(k_r/J_Pzz - (R_m*d_P + K_g*eta_g*eta_m*k_b*k_m)^2/(J_Pzz^2*R_m^2)) - p3*(((k_r/J_Pzz - (R_m*d_P + K_g*eta_g*eta_m*k_b*k_m)^2/(J_Pzz^2*R_m^2))*(R_m*d_P + K_g*eta_g*eta_m*k_b*k_m))/(J_Pzz*R_m) + (k_r*(R_m*d_P + K_g*eta_g*eta_m*k_b*k_m))/(J_Pzz^2*R_m)) - p0 + (k_r*((R_m*d_P + K_g*eta_g*eta_m*k_b*k_m)^2/(J_Pzz^2*R_m^2) - (k_r*(J_Bzz + J_Pzz))/(J_Bzz*J_Pzz)))/J_Pzz + (p1*(R_m*d_P + K_g*eta_g*eta_m*k_b*k_m))/(J_Pzz*R_m) + ((((k_r/J_Pzz - (R_m*d_P + K_g*eta_g*eta_m*k_b*k_m)^2/(J_Pzz^2*R_m^2))*(R_m*d_P + K_g*eta_g*eta_m*k_b*k_m))/(J_Pzz*R_m) + (k_r*(R_m*d_P + K_g*eta_g*eta_m*k_b*k_m))/(J_Pzz^2*R_m))*(R_m*d_P + K_g*eta_g*eta_m*k_b*k_m))/(J_Pzz*R_m)))/k_r;
    l(3,1) = -(J_Bzz*(p1 + p3*((R_m*d_P + K_g*eta_g*eta_m*k_b*k_m)^2/(J_Pzz^2*R_m^2) - (k_r*(J_Bzz + J_Pzz))/(J_Bzz*J_Pzz)) + ((k_r/J_Pzz - (R_m*d_P + K_g*eta_g*eta_m*k_b*k_m)^2/(J_Pzz^2*R_m^2))*(R_m*d_P + K_g*eta_g*eta_m*k_b*k_m))/(J_Pzz*R_m) + (((k_r*(J_Bzz + J_Pzz))/(J_Bzz*J_Pzz) - (g*l_G*cos(x1 + x3)*(m_B1 + m_B2))/J_Bzz)*(R_m*d_P + K_g*eta_g*eta_m*k_b*k_m))/(J_Pzz*R_m) - (p2*(R_m*d_P + K_g*eta_g*eta_m*k_b*k_m))/(J_Pzz*R_m) + (g*l_G*cos(x1 + x3)*(m_B1 + m_B2)*(R_m*d_P + K_g*eta_g*eta_m*k_b*k_m))/(J_Bzz*J_Pzz*R_m)))/k_r;
    l(4,1) = -(J_Bzz*(p0 + p2*((R_m*d_P + K_g*eta_g*eta_m*k_b*k_m)^2/(J_Pzz^2*R_m^2) - (k_r*(J_Bzz + J_Pzz))/(J_Bzz*J_Pzz)) - ((k_r*(J_Bzz + J_Pzz))/(J_Bzz*J_Pzz) - (g*l_G*cos(x1 + x3)*(m_B1 + m_B2))/J_Bzz)*((R_m*d_P + K_g*eta_g*eta_m*k_b*k_m)^2/(J_Pzz^2*R_m^2) - (k_r*(J_Bzz + J_Pzz))/(J_Bzz*J_Pzz)) + p3*(((k_r/J_Pzz - (R_m*d_P + K_g*eta_g*eta_m*k_b*k_m)^2/(J_Pzz^2*R_m^2))*(R_m*d_P + K_g*eta_g*eta_m*k_b*k_m))/(J_Pzz*R_m) + (((k_r*(J_Bzz + J_Pzz))/(J_Bzz*J_Pzz) - (g*l_G*cos(x1 + x3)*(m_B1 + m_B2))/J_Bzz)*(R_m*d_P + K_g*eta_g*eta_m*k_b*k_m))/(J_Pzz*R_m) + (g*l_G*cos(x1 + x3)*(m_B1 + m_B2)*(R_m*d_P + K_g*eta_g*eta_m*k_b*k_m))/(J_Bzz*J_Pzz*R_m)) - (p1*(R_m*d_P + K_g*eta_g*eta_m*k_b*k_m))/(J_Pzz*R_m) - ((((k_r/J_Pzz - (R_m*d_P + K_g*eta_g*eta_m*k_b*k_m)^2/(J_Pzz^2*R_m^2))*(R_m*d_P + K_g*eta_g*eta_m*k_b*k_m))/(J_Pzz*R_m) + (k_r*(R_m*d_P + K_g*eta_g*eta_m*k_b*k_m))/(J_Pzz^2*R_m))*(R_m*d_P + K_g*eta_g*eta_m*k_b*k_m))/(J_Pzz*R_m) + (g*l_G*cos(x1 + x3)*(m_B1 + m_B2)*(k_r/J_Pzz - (R_m*d_P + K_g*eta_g*eta_m*k_b*k_m)^2/(J_Pzz^2*R_m^2)))/J_Bzz))/k_r;
    y_est = x_est(1) + x_est(3);
    y_ref = x_ref(1) + x_ref(3);
    delta_y_est = y_est - y_ref;

    delta_x_est_dot = f_x_est - f_x_ref + gx*delta_u + l*(delta_y - delta_y_est);
end
